simulink model "ExperimentSSNominalModelDirectDigital"  (R2020b)
settings: Solver=FixedStepDiscrete  StartTime=0.0  StopTime=10  FixedStep=Ts  RelTol=1e-3
undefined symbols (not defined in the file): finalValue, Gamma0, H0, J0, K, National_Instruments, Nu, Nx, PCI, Phi0, sens, Ts
libraries: sldrtlib x3
settings Model: ExtModeTrigDuration=100000  Creator=umbe  LastModifiedBy=Diego
settings DataIOCC: ReturnWorkspaceOutputs=off
settings RTWCC: Description=Simulink Desktop Real-Time  SystemTargetFile=sldrt.tlc  TemplateMakefile=sldrt.tmf  RTWCompilerOptimization=on
settings CodeAppCC: MaxIdLength=95
settings SimulinkDesktopRealTimeCC: TargetPreCompLibLocation=C:\Program Files\MATLAB\R2020b\toolbox\sldrt\lib\win64

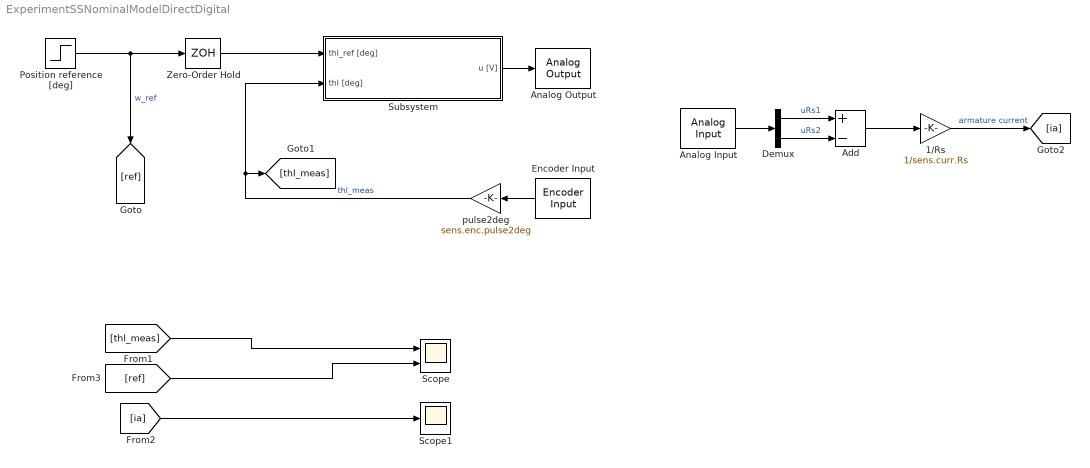
== system ExperimentSSNominalModelDirectDigital ==
  1/Rs : Gain  Gain=1/sens.curr.Rs
  Add : Sum  Inputs=+-
  Analog Input : sldrtlib/Analog Input  SampleTime=Ts  MaxMissedTicks=10  ShowMissedTicks=off  YieldWhenWaiting=off  DrvName=National_Instruments/PCI-6221  DrvAddress=4294967295  DrvOptions=[0 0 0 2 0]  Channels=[1 2]  RangeMode=1  VoltRange=1  DataType=1
      settings: AttributesFormatString=National Instruments\nPCI-6221 [auto]
  Analog Output : sldrtlib/Analog Output  SampleTime=Ts  MaxMissedTicks=10  ShowMissedTicks=off  YieldWhenWaiting=off  DrvName=National_Instruments/PCI-6221  DrvAddress=4294967295  DrvOptions=[0 0 0 2 0]  Channels=1  RangeMode=1  VoltRange=1  InitialValue=0  FinalValue=0
      settings: AttributesFormatString=National Instruments\nPCI-6221 [auto]
  Demux : Demux  Outputs=2
  Encoder Input : sldrtlib/Encoder Input  SampleTime=Ts  MaxMissedTicks=10  ShowMissedTicks=off  YieldWhenWaiting=off  DrvName=National_Instruments/PCI-6221  DrvAddress=4294967295  DrvOptions=[0 0 0 2 0]  Channels=1  QuadMode=3  IndexPulse=1  InputFilter=Inf  DataType=1
      settings: AttributesFormatString=National Instruments\nPCI-6221 [auto]
  Position reference [deg] : Step  After=finalValue  SampleTime=0
  Scope : Scope  NumInputPorts=2
  Scope1 : Scope
  Subsystem : Subsystem
  Zero-Order Hold : ZeroOrderHold  SampleTime=Ts
  pulse2deg : Gain  Gain=sens.enc.pulse2deg
  wires:
  1/Rs/1 -> [ia]  "armature current"
  Add/1 -> 1/Rs/1
  Demux/1 -> Add/1  "uRs1"
  Demux/2 -> Add/2  "uRs2"
  pulse2deg/1 -> Subsystem/2(thl [deg]), [thl_meas]  "thl_meas"
  [thl_meas] -> Scope/1
  [ia] -> Scope1/1
  Encoder Input/1 -> pulse2deg/1
  Analog Input/1 -> Demux/1
  Subsystem/1(u [V]) -> Analog Output/1
  Position reference [deg]/1 -> [ref], Zero-Order Hold/1  "w_ref"
  Zero-Order Hold/1 -> Subsystem/1(thl_ref [deg])
  [ref] -> Scope/2

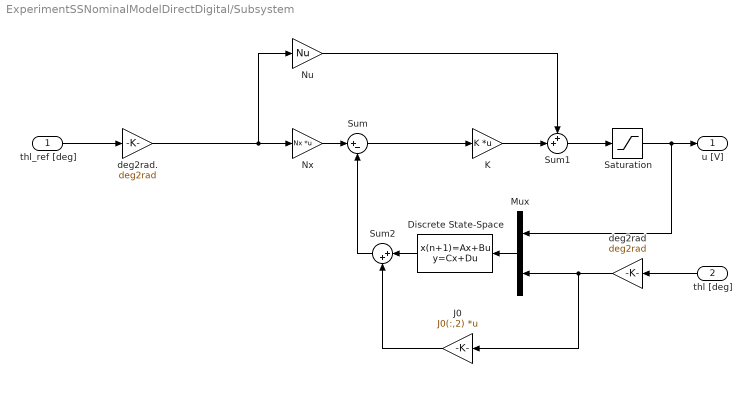
== system ExperimentSSNominalModelDirectDigital/Subsystem ==
  thl_ref [deg] : Inport
  thl [deg] : Inport  Port=2
  Discrete State-Space : DiscreteStateSpace  A=Phi0  B=Gamma0  C=H0  D=zeros(size(H0,1),size(Gamma0,2))  SampleTime=Ts
  J0 : Gain  Gain=J0(:,2)  Multiplication=Matrix(K*u)
  K : Gain  Gain=K  Multiplication=Matrix(K*u)
  Mux : Mux  Inputs=2
  Nu : Gain  Gain=Nu
  Nx : Gain  Gain=Nx  Multiplication=Matrix(K*u)
  Saturation : Saturate  UpperLimit=10  LowerLimit=-10
  Sum : Sum  Inputs=|+-
  Sum1 : Sum  Inputs=++|
  Sum2 : Sum  Inputs=|++
  deg2rad : Gain  Gain=deg2rad
  deg2rad. : Gain  Gain=deg2rad
  u [V] : Outport
  wires:
  deg2rad/1 -> J0/1, Mux/2
  thl [deg]/1 -> deg2rad/1
  Saturation/1 -> Mux/1, u [V]/1
  thl_ref [deg]/1 -> deg2rad./1
  deg2rad./1 -> Nx/1, Nu/1
  Nx/1 -> Sum/1
  Mux/1 -> Discrete State-Space/1
  Sum/1 -> K/1
  K/1 -> Sum1/2
  Nu/1 -> Sum1/1
  Sum1/1 -> Saturation/1
  Discrete State-Space/1 -> Sum2/1
  J0/1 -> Sum2/2
  Sum2/1 -> Sum/2
